simulink model "Aufgabe_5_2_2_Temperaturregelung"  (R2023b)
settings: Solver=VariableStepAuto  StartTime=0.0  StopTime=10.0  RelTol=1e-3
undefined symbols (not defined in the file or in its folder): sigbuilder_block
settings Model: Creator=JCP  LastModifiedBy=JCP

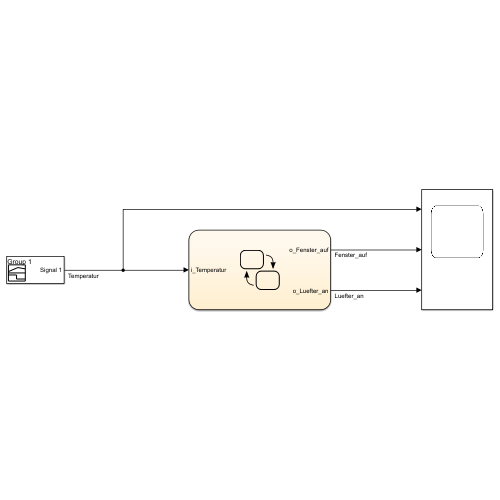
[thumbnail: Simulink's stored preview of the top-level diagram]
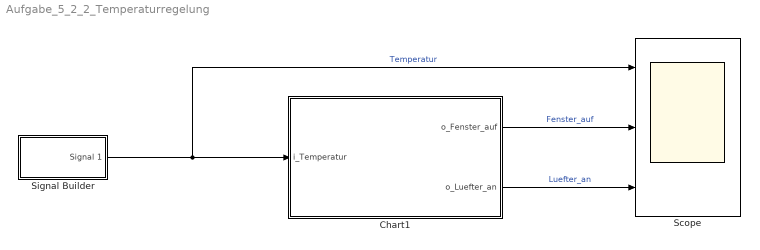
== system Aufgabe_5_2_2_Temperaturregelung ==
  Chart1 : Stateflow chart  TreatAsAtomicUnit=on
  Scope : Scope  NumInputPorts=3
  Signal Builder : Subsystem  Tag=STV Subsys  LoadFcn=sigbuilder_block('load');  StartFcn=sigbuilder_block('start');  StopFcn=sigbuilder_block('stop');  ClipboardFcn=sigbuilder_block('clipboard');  mask(Sigbuilder block){tuvar=[0:10]}
      mask help: Simulink:masks:SigbuilderBlock_MD
      mask init:
      | if ~strcmp(get_param(bdroot(gcbh),'SimulationStatus'),'stopped') tuvar = sigbuilder_block('maskInit'); end
      settings: CopyFcn=sigbuilder_block('copy');  DeleteFcn=sigbuilder_block('delete');  ModelCloseFcn=sigbuilder_block('modelClose');  PreSaveFcn=sigbuilder_block('preSave');  PauseFcn=sigbuilder_block('pause');  ContinueFcn=sigbuilder_block('continue');  NameChangeFcn=sigbuilder_block('namechange');  OpenFcn=sigbuilder_block('open',[231 84.75 550.5 395.25 ]);  CloseFcn=sigbuilder_block('close');
      mask Display: plot(0, 0, 100, 100,[2, 2, 32, 32, 2], [68, 8, 8, 68, 68],[32, 2], [38, 38], [32, 19, 2],[53, 60, 44], [32, 17, 17, 2],[16, 16, 31, 31]);txt = getActiveGroup(gcbh);text(2, 100, txt,'verticalAlignment', 'top');
  wires:
  Signal Builder/1(Signal 1) -> Scope/1, Chart1/1(i_Temperatur)  "Temperatur"
  Chart1/1(o_Fenster_auf) -> Scope/2  "Fenster_auf"
  Chart1/2(o_Luefter_an) -> Scope/3  "Luefter_an"

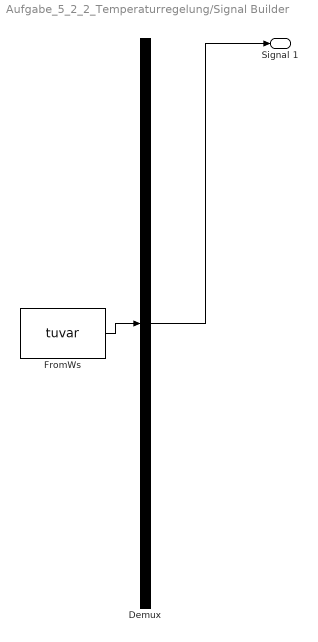
== system Aufgabe_5_2_2_Temperaturregelung/Signal Builder ==
  Demux : Demux  Tag=STV Demux  Outputs=1
      settings: DisplayOption=none
  FromWs : FromWorkspace  Tag=STV FromWs  VariableName=tuvar
      SigBuilderData=|
      | common.afterFinalStr = 'Extrapolate'
      | common.sampleTime = 0
      | dataSet.timeRange = [0 40]
      | dataSet.name = 'Group 1'
      | sbobj.Groups.Name = 'Group 1'
      | sbobj.Groups.Signals.Name = 'Signal 1'
      | sbobj.Groups.Signals.XData = [0 5 10 15 22 28.2 40]
      | sbobj.Groups.Signals.YData = [20 28 19 32 23 32 18]
      | sbobj.Groups.TimeRange = [0 40]
  Signal 1 : Outport  Tag=STV Outport
  wires:
  Demux/1 -> Signal 1/1
  FromWs/1 -> Demux/1

== stateflow chart Aufgabe_5_2_2_Temperaturregelung/Chart1 ==
  state Fenster [parallel]
    settings: executionOrder=1
    state Fenster_zu
      en: o_Fenster_auf =0;
    state Fenster_offen
      en: o_Fenster_auf = 1;
    (default) -> Fenster_zu
    Fenster_zu -> Fenster_offen : [i_Temperatur >25]
    Fenster_offen -> Fenster_zu : [i_Temperatur<20]
  state Luefter [parallel]
    settings: executionOrder=2
    state Luefter_zu
      en: o_Luefter_an = 0;
    state Luefter_offen
      en: o_Luefter_an = 1;
    (default) -> Luefter_zu
    Luefter_zu -> Luefter_offen : [i_Temperatur >30]
    Luefter_offen -> Luefter_zu : [i_Temperatur <25]
  data: o_Fenster_auf output; o_Luefter_an output; i_Temperatur input
